simulink model "grid_connected_induction_generator"  (R2014b)
settings: Solver=ode23tb  StartTime=0.0  StopTime=1000  MaxStep=1e-4  RelTol=1e-3
libraries: powerlib x8, simulink x1
settings Model: Creator=Amr Saleh  LastModifiedBy=Amr Saleh

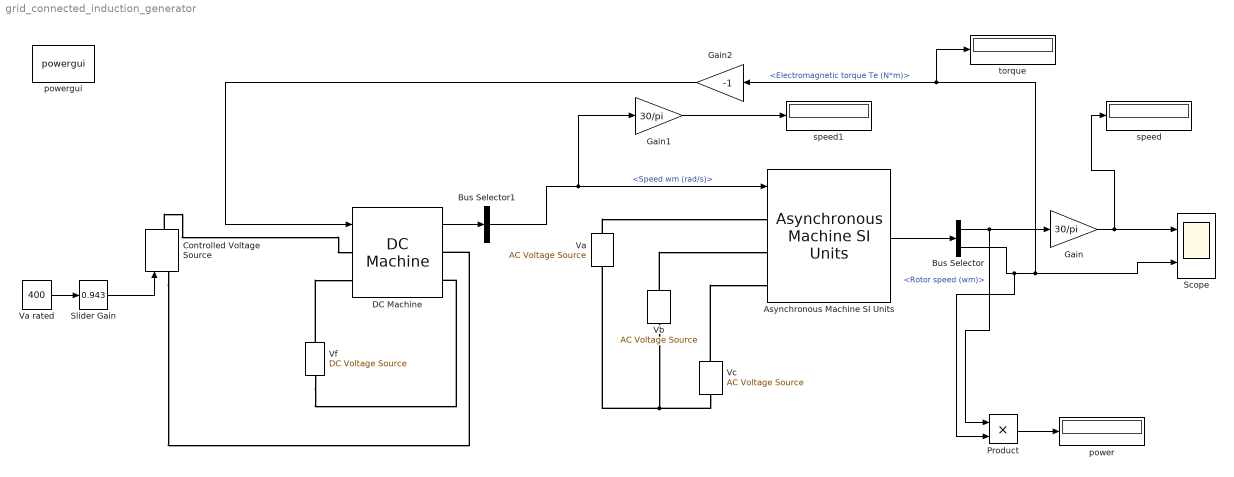
== system grid_connected_induction_generator ==
  Asynchronous Machine SI Units : powerlib/Machines/Asynchronous Machine SI Units  PresetModel="15:  5.4 HP (4KW)   400 V  50Hz 1430 RPM"  MechanicalLoad=Speed w  ShowDetailedParameters=on  RotorType=Squirrel-cage  ReferenceFrame=Stationary  Units=SI  MeasurementBus=off  NominalParameters=[4000 400 50]  Stator=[1.405 0.005839]  Rotor=[1.395 0.005839]  Cage1=[ 0.022 0.226/377]  Cage2=[ 0.022 0.226/377]  Lm=0.1722  Mechanical=[0.0131 0.002985 2]  PolePairs=2  InitialConditions=[1 0 0 0 0 0 0 0]  SimulateSaturation=off  Saturation=[14.03593122, 27.81365428, 53.79336849, 72.68890987, 97.98006896, 148.6815601, 215.7428561, 302.9841135, 420.4778367 ; 230, 322, 414, 460, 506, 552, 598, 644, 690]  LoadFlowParameters=1492000  TsPowergui=0  TsBlock=-1  IterativeModel=Trapezoidal non iterative  Pmec=0
  Bus Selector : BusSelector  OutputSignals=Mechanical.Rotor speed (wm),Mechanical.Electromagnetic torque Te (N*m)
  Bus Selector1 : BusSelector  OutputSignals=Speed wm (rad/s)
  Controlled Voltage Source : powerlib/Electrical Sources/Controlled Voltage Source  Initialize=on  Source_Type=AC  Amplitude=0  Phase=0  Frequency=0  Measurements=None
  DC Machine : powerlib/Machines/DC Machine  PresetModel=No  MechanicalLoad=Torque TL  FieldType=Wound  ShowDetailedParameters=on  MeasurementBus=off  RLa="[ 0.6  0.012]"  RLf="[ 240  120]"  Laf=1.8  MachineConstant=Torque constant (N.m/A)  Ke=1.8  Kt=1.8  J=1  Bm=0  Tf=0  w0=1  Ifinit=1  TsPowergui=0  TsBlock=-1
  Gain : Gain  Gain=30/pi
  Gain1 : Gain  Gain=30/pi
  Gain2 : Gain  Gain=-1
  Product : Product
  Scope : Scope  NumInputPorts=2
      settings: YMin=-5~-5  YMax=5~5
  Slider Gain : simulink/Math Operations/Slider Gain  low=0  gain=0.943  high=1
  Va : powerlib/Electrical Sources/AC Voltage Source  Amplitude=326  Phase=0  Frequency=50  SampleTime=0  Measurements=None
  Va rated : Constant  Value=400
  Vb : powerlib/Electrical Sources/AC Voltage Source  Amplitude=326  Phase=-120  Frequency=50  SampleTime=0  Measurements=None
  Vc : powerlib/Electrical Sources/AC Voltage Source  Amplitude=326  Phase=120  Frequency=50  SampleTime=0  Measurements=None
  Vf : powerlib/Electrical Sources/DC Voltage Source  Amplitude=300  Measurements=None
  power : Display
  powergui : powerlib/powergui  Priority=1  SimulationMode=Continuous  SolverType=Tustin/Backward Euler (TBE)  SampleTime=50e-6  frequency=60  SPID=off  DisableSnubberDevices=off  DisableRonSwitches=off  DisableVfSwitches=off  SwTol=0  DisplayEquations=off  Interpol=off  methode=off  Ts=100  frequencyindice=0  Pbase=100e6  ErrMax=1e-4  Iterations=50  UnitsV=kV  UnitsW=MW  FunctionMessages=off  echomessages=off  HookPort=off  EnableUseOfTLC=off  x0status=blocks  RestoreLinks=warning  ResistiveCurrentMeasurement=off  Frange=[0:2:500]  Ylog=off  Xlog=on  ShowGrid=off  save=off  variable=ZData  structure=0  ZoomFFT=off  StartTime=0.0  cycles=1  DisplayStyle=1  fundamental=60  FreqAxis=off  MaxFrequency=1000  frequencyindicesteady=1  RmsSteady=1  display=off
  speed : Display
  speed1 : Display
  torque : Display
  wires:
  Asynchronous Machine SI Units/1 -> Bus Selector/1
  Bus Selector/1 -> Product/1, Gain/1  "<Rotor speed (wm)>"
  Gain/1 -> speed/1, Scope/1
  Bus Selector/2 -> Product/2, torque/1, Gain2/1, Scope/2  "<Electromagnetic torque Te (N*m)>"
  DC Machine/1 -> Bus Selector1/1
  Bus Selector1/1 -> Asynchronous Machine SI Units/1, Gain1/1  "<Speed wm (rad/s)>"
  Gain1/1 -> speed1/1
  Va rated/1 -> Slider Gain/1
  Slider Gain/1 -> Controlled Voltage Source/1
  Gain2/1 -> DC Machine/1
  Product/1 -> power/1
  connections:
  Va/RConn1 -- Asynchronous Machine SI Units/LConn1
  Vb/RConn1 -- Asynchronous Machine SI Units/LConn2
  Vc/RConn1 -- Asynchronous Machine SI Units/LConn3
  Vc/LConn1 -- Va/LConn1 -- Vb/LConn1
  Vf/RConn1 -- DC Machine/LConn2
  Vf/LConn1 -- DC Machine/RConn2
  Controlled Voltage Source/RConn1 -- DC Machine/LConn1
  Controlled Voltage Source/LConn1 -- DC Machine/RConn1
